simulink model "RTinductionmotor2017blatest"  (R2017b)
settings: Solver=VariableStepAuto  StartTime=0.0  StopTime=0.25  RelTol=1e-3
libraries: powerlib_meascontrol x1
settings Model: Creator=adam_  LastModifiedBy=adam_
settings DataIOCC: ReturnWorkspaceOutputs=on
settings SFSimCC: SimUseLocalCustomCode=on
settings RTWCC: RTWUseLocalCustomCode=on

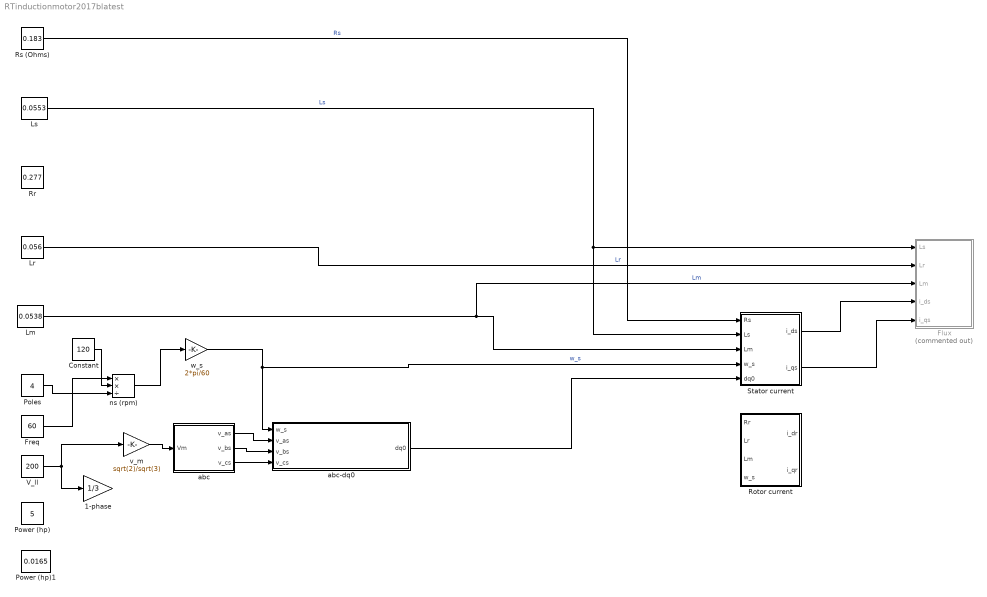
== system RTinductionmotor2017blatest ==
  1-phase : Gain  Gain=1/3
  Constant : Constant  Value=120
  Flux : Subsystem  Commented=on
  Freq : Constant  Value=60
  "Lm " : Constant  Value=0.0538
  Lr : Constant  Value=0.056
  "Ls " : Constant  Value=0.0553
  Poles : Constant  Value=4
  Power (hp) : Constant  Value=5
  Power (hp)1 : Constant  Value=0.0165
  Rotor current : Subsystem
  "Rr " : Constant  Value=0.277
  Rs (Ohms) : Constant  Value=0.183
  Stator current : Subsystem
  V_ll : Constant  Value=200
  abc : Subsystem
  abc-dq0 : Subsystem
  ns (rpm) : Product  Inputs=**/
  v_m : Gain  Gain=sqrt(2)/sqrt(3)
  w_s : Gain  Gain=2*pi/60
  wires:
  V_ll/1 -> v_m/1, 1-phase/1
  Freq/1 -> ns (rpm)/1
  Poles/1 -> ns (rpm)/3
  Constant/1 -> ns (rpm)/2
  abc/1(v_as) -> abc-dq0/2(v_as)
  abc/2(v_bs) -> abc-dq0/3(v_bs)
  abc/3(v_cs) -> abc-dq0/4(v_cs)
  ns (rpm)/1 -> w_s/1
  w_s/1 -> Stator current/4(w_s), abc-dq0/1(w_s)  "w_s"
  v_m/1 -> abc/1(Vm)
  Rs (Ohms)/1 -> Stator current/1(Rs)  "Rs"
  "Ls "/1 -> Stator current/2(Ls), Flux/1(Ls)  "Ls"
  "Lm "/1 -> Flux/3(Lm), Stator current/3(Lm)  "Lm"
  abc-dq0/1(dq0) -> Stator current/5(dq0)
  Stator current/1(i_ds) -> Flux/4(i_ds)
  Stator current/2(i_qs) -> Flux/5(i_qs)
  Lr/1 -> Flux/2(Lr)  "Lr"

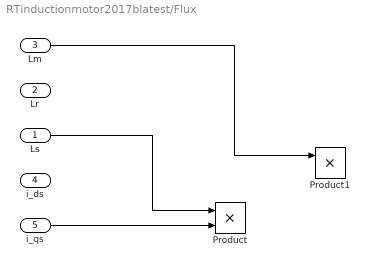
== system RTinductionmotor2017blatest/Flux ==
  Ls : Inport
  Lr : Inport  Port=2
  Lm : Inport  Port=3
  i_ds : Inport  Port=4
  i_qs : Inport  Port=5
  Product : Product
  Product1 : Product
  wires:
  Ls/1 -> Product/1
  i_qs/1 -> Product/2
  Lm/1 -> Product1/1

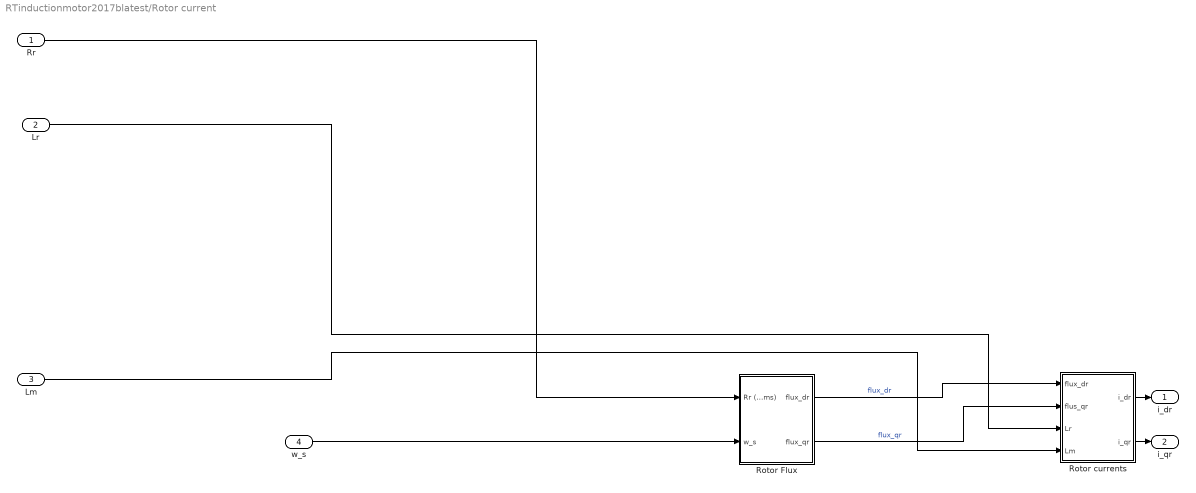
== system RTinductionmotor2017blatest/Rotor current ==
  Rr : Inport
  Lr : Inport  Port=2
  Lm : Inport  Port=3
  w_s : Inport  Port=4
  Rotor Flux : Subsystem
  Rotor currents : Subsystem
  i_dr : Outport
  i_qr : Outport  Port=2
  wires:
  Rotor Flux/2(flux_qr) -> Rotor currents/2(flus_qr)  "flux_qr"
  Rotor Flux/1(flux_dr) -> Rotor currents/1(flux_dr)  "flux_dr"
  Rr/1 -> Rotor Flux/1(Rr (Ohms))
  Lr/1 -> Rotor currents/3(Lr)
  Lm/1 -> Rotor currents/4(Lm)
  Rotor currents/1(i_dr) -> i_dr/1
  w_s/1 -> Rotor Flux/2(w_s)
  Rotor currents/2(i_qr) -> i_qr/1

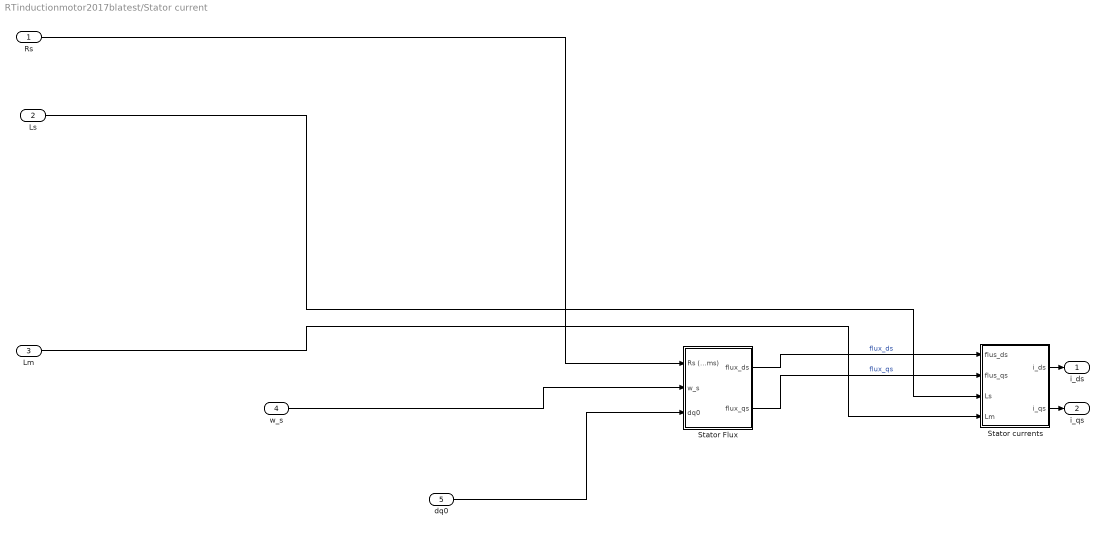
== system RTinductionmotor2017blatest/Stator current ==
  Rs : Inport
  Ls : Inport  Port=2
  Lm : Inport  Port=3
  w_s : Inport  Port=4
  dq0 : Inport  Port=5
  Stator Flux : Subsystem
  Stator currents : Subsystem
  i_ds : Outport
  i_qs : Outport  Port=2
  wires:
  Stator Flux/2(flux_qs) -> Stator currents/2(flus_qs)  "flux_qs"
  Stator Flux/1(flux_ds) -> Stator currents/1(flus_ds)  "flux_ds"
  Rs/1 -> Stator Flux/1(Rs (Ohms))
  Ls/1 -> Stator currents/3(Ls)
  Lm/1 -> Stator currents/4(Lm)
  Stator currents/1(i_ds) -> i_ds/1
  w_s/1 -> Stator Flux/2(w_s)
  Stator currents/2(i_qs) -> i_qs/1
  dq0/1 -> Stator Flux/3(dq0)

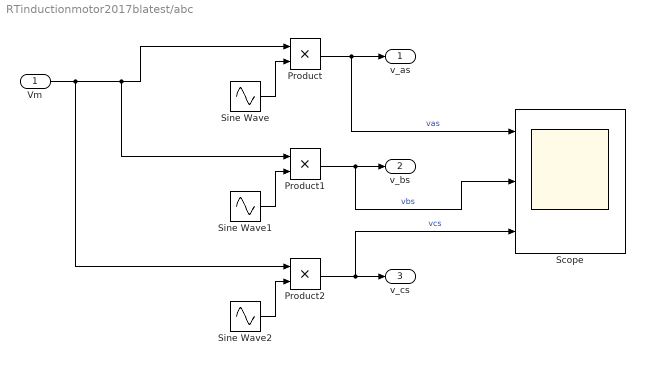
== system RTinductionmotor2017blatest/abc ==
  Vm : Inport
  Product : Product
  Product1 : Product
  Product2 : Product
  Scope : Scope  NumInputPorts=3
  Sine Wave : Sin  Frequency=60*2*pi  SampleTime=0.0001  VectorParams1D=off
  Sine Wave1 : Sin  Frequency=60*2*pi  Phase=-2*pi/3  SampleTime=0.0001  VectorParams1D=off
  Sine Wave2 : Sin  Frequency=60*2*pi  Phase=2*pi/3  SampleTime=0.0001  VectorParams1D=off
  v_as : Outport
  v_bs : Outport  Port=2
  v_cs : Outport  Port=3
  wires:
  Sine Wave/1 -> Product/2
  Product/1 -> Scope/1, v_as/1  "vas"
  Product1/1 -> Scope/2, v_bs/1  "vbs"
  Sine Wave1/1 -> Product1/2
  Product2/1 -> Scope/3, v_cs/1  "vcs"
  Vm/1 -> Product2/1, Product1/1, Product/1
  Sine Wave2/1 -> Product2/2

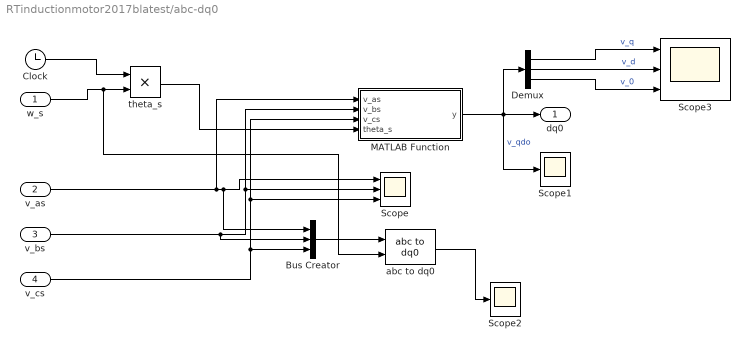
== system RTinductionmotor2017blatest/abc-dq0 ==
  w_s : Inport
  v_as : Inport  Port=2
  v_bs : Inport  Port=3
  v_cs : Inport  Port=4
  Bus Creator : BusCreator  Inputs=3
  Clock : Clock
  Demux : Demux  Outputs=3
  MATLAB Function : MATLAB Function  TreatAsAtomicUnit=on
  Scope : Scope  NumInputPorts=3
  Scope1 : Scope
  Scope2 : Scope
  Scope3 : Scope  NumInputPorts=3
  abc to dq0 : powerlib_meascontrol/Transformations/abc to dq0  Alignment=90 degrees behind phase A axis
  theta_s : Product
  dq0 : Outport
  wires:
  v_as/1 -> MATLAB Function/1(v_as), Bus Creator/1, Scope/1
  v_cs/1 -> Bus Creator/3, Scope/3, MATLAB Function/3(v_cs)
  MATLAB Function/1(y) -> Demux/1, Scope1/1, dq0/1  "v_qdo"
  v_bs/1 -> Bus Creator/2, Scope/2, MATLAB Function/2(v_bs)
  w_s/1 -> abc to dq0/2, theta_s/2
  Clock/1 -> theta_s/1
  theta_s/1 -> MATLAB Function/4(theta_s)
  Bus Creator/1 -> abc to dq0/1
  abc to dq0/1 -> Scope2/1
  Demux/1 -> Scope3/1  "v_q"
  Demux/2 -> Scope3/2  "v_d"
  Demux/3 -> Scope3/3  "v_0"

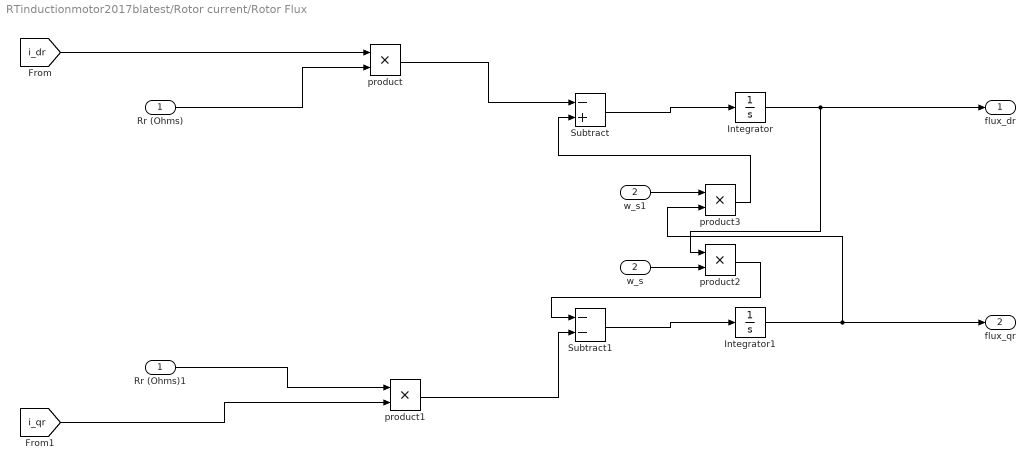
== system RTinductionmotor2017blatest/Rotor current/Rotor Flux ==
  Rr (Ohms) : Inport
  w_s : Inport  Port=2
  Integrator : Integrator
  Integrator1 : Integrator
  Rr (Ohms)1 : InportShadow
  Subtract : Sum  Inputs=-+
  Subtract1 : Sum  Inputs=--
  product{,1..3} (4 alike) : Product  Inputs=**
  w_s1 : InportShadow  Port=2
  flux_dr : Outport  VectorParamsAs1DForOutWhenUnconnected=off
  flux_qr : Outport  Port=2  VectorParamsAs1DForOutWhenUnconnected=off
  wires:
  Rr (Ohms)/1 -> product/2
  product/1 -> Subtract/1
  Subtract/1 -> Integrator/1
  Integrator/1 -> product2/1, flux_dr/1
  Subtract1/1 -> Integrator1/1
  product1/1 -> Subtract1/2
  [i_dr] -> product/1
  Integrator1/1 -> product3/2, flux_qr/1
  Rr (Ohms)1/1 -> product1/1
  w_s1/1 -> product3/1
  product3/1 -> Subtract/2
  w_s/1 -> product2/2
  product2/1 -> Subtract1/1
  [i_qr] -> product1/2

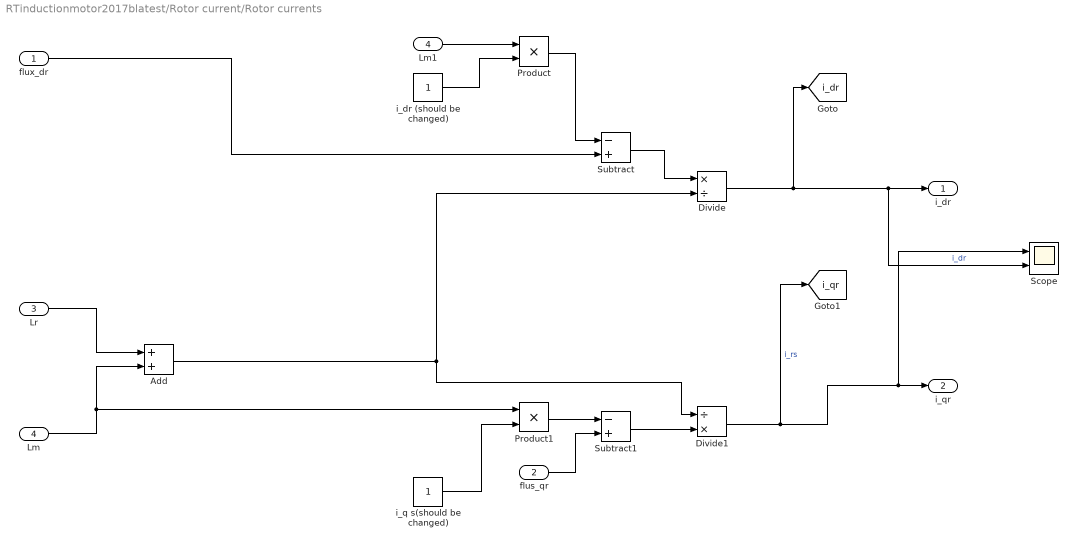
== system RTinductionmotor2017blatest/Rotor current/Rotor currents ==
  flux_dr : Inport
  flus_qr : Inport  Port=2
  Lr : Inport  Port=3
  Lm : Inport  Port=4
  Add : Sum
  Divide : Product  Inputs=*/
  Divide1 : Product  Inputs=/*
  Lm1 : InportShadow  Port=4
  Product : Product
  Product1 : Product
  Scope : Scope  NumInputPorts=2
  Subtract : Sum  Inputs=-+
  Subtract1 : Sum  Inputs=-+
  i_dr (should be changed) : Constant
  i_q s(should be changed) : Constant
  i_dr : Outport  VectorParamsAs1DForOutWhenUnconnected=off
  i_qr : Outport  Port=2  VectorParamsAs1DForOutWhenUnconnected=off
  tag scope: i_dr=global, i_qr=global
  wires:
  Lm1/1 -> Product/1
  i_dr (should be changed)/1 -> Product/2
  flux_dr/1 -> Subtract/2
  Product/1 -> Subtract/1
  Lr/1 -> Add/1
  Lm/1 -> Product1/1, Add/2
  Subtract/1 -> Divide/1
  Add/1 -> Divide1/1, Divide/2
  Divide/1 -> [i_dr], Scope/2, i_dr/1  "i_dr"
  i_q s(should be changed)/1 -> Product1/2
  Product1/1 -> Subtract1/1
  flus_qr/1 -> Subtract1/2
  Subtract1/1 -> Divide1/2
  Divide1/1 -> [i_qr], Scope/1, i_qr/1  "i_rs"

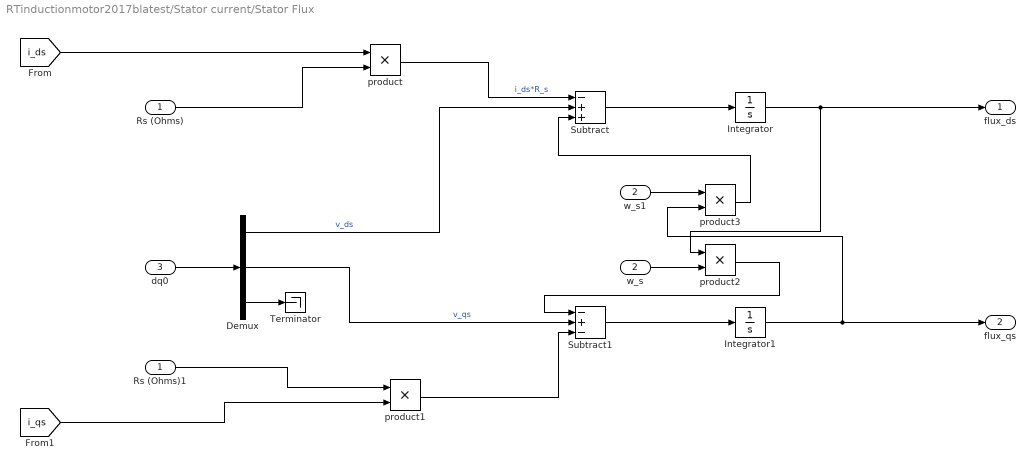
== system RTinductionmotor2017blatest/Stator current/Stator Flux ==
  Rs (Ohms) : Inport
  w_s : Inport  Port=2
  dq0 : Inport  Port=3
  Demux : Demux  Outputs=3
  Integrator : Integrator
  Integrator1 : Integrator
  Rs (Ohms)1 : InportShadow
  Subtract : Sum  Inputs=-++
  Subtract1 : Sum  Inputs=-+-
  Terminator : Terminator
  product{,1..3} (4 alike) : Product  Inputs=**
  w_s1 : InportShadow  Port=2
  flux_ds : Outport  VectorParamsAs1DForOutWhenUnconnected=off
  flux_qs : Outport  Port=2  VectorParamsAs1DForOutWhenUnconnected=off
  wires:
  dq0/1 -> Demux/1
  Demux/3 -> Terminator/1
  Rs (Ohms)/1 -> product/2
  product/1 -> Subtract/1  "i_ds*R_s"
  Demux/1 -> Subtract/2  "v_ds"
  Subtract/1 -> Integrator/1
  Integrator/1 -> product2/1, flux_ds/1
  Subtract1/1 -> Integrator1/1
  product1/1 -> Subtract1/3
  [i_ds] -> product/1
  Demux/2 -> Subtract1/2  "v_qs"
  Integrator1/1 -> product3/2, flux_qs/1
  Rs (Ohms)1/1 -> product1/1
  w_s1/1 -> product3/1
  product3/1 -> Subtract/3
  w_s/1 -> product2/2
  product2/1 -> Subtract1/1
  [i_qs] -> product1/2

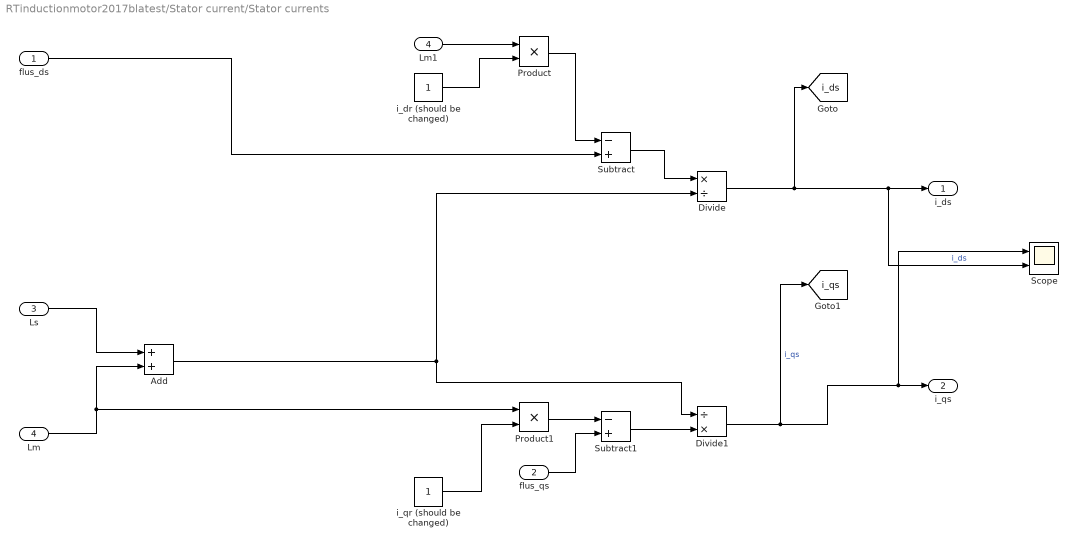
== system RTinductionmotor2017blatest/Stator current/Stator currents ==
  flus_ds : Inport
  flus_qs : Inport  Port=2
  Ls : Inport  Port=3
  Lm : Inport  Port=4
  Add : Sum
  Divide : Product  Inputs=*/
  Divide1 : Product  Inputs=/*
  Lm1 : InportShadow  Port=4
  Product : Product
  Product1 : Product
  Scope : Scope  NumInputPorts=2
  Subtract : Sum  Inputs=-+
  Subtract1 : Sum  Inputs=-+
  i_dr (should be changed) : Constant
  i_qr (should be changed) : Constant
  i_ds : Outport  VectorParamsAs1DForOutWhenUnconnected=off
  i_qs : Outport  Port=2  VectorParamsAs1DForOutWhenUnconnected=off
  tag scope: i_ds=global, i_qs=global
  wires:
  Lm1/1 -> Product/1
  i_dr (should be changed)/1 -> Product/2
  flus_ds/1 -> Subtract/2
  Product/1 -> Subtract/1
  Ls/1 -> Add/1
  Lm/1 -> Product1/1, Add/2
  Subtract/1 -> Divide/1
  Add/1 -> Divide1/1, Divide/2
  Divide/1 -> [i_ds], Scope/2, i_ds/1  "i_ds"
  i_qr (should be changed)/1 -> Product1/2
  Product1/1 -> Subtract1/1
  flus_qs/1 -> Subtract1/2
  Subtract1/1 -> Divide1/2
  Divide1/1 -> [i_qs], Scope/1, i_qs/1  "i_qs"

== matlab function RTinductionmotor2017blatest/abc-dq0/MATLAB Function ==
  data: v_as input; y output; v_bs input; v_cs input; theta_s input
function y = fcn(v_as, v_bs, v_cs, theta_s)
%#codegen
T_abc = 2/3 * ...
    [ cos(theta_s) cos(theta_s-(2*pi/3)) cos(theta_s + (2*pi/3));...
    sin(theta_s) sin(theta_s-(2*pi/3)) sin(theta_s + (2*pi/3));...
    1/2 1/2 1/2 ];
v_abc = [ v_as;v_bs;v_cs] ; 
v_qdo = T_abc * v_abc ;
y = v_qdo;
